simulink model "ModelStepper"  (R2020b)
settings: Solver=FixedStepAuto  StartTime=0.0  StopTime=10.0  FixedStep=0.010  RelTol=1e-3
settings Model: Creator=kaebi  LastModifiedBy=kaebi
settings ConfigComp: PLC_TargetIDE=codesys23

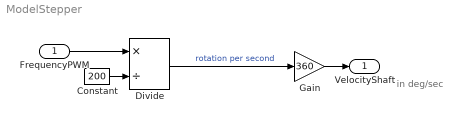
== system ModelStepper ==
  note: in deg/sec
  FrequencyPWM : Inport
  Constant : Constant  Value=200
  Divide : Product  Inputs=*/
  Gain : Gain  Gain=360
  VelocityShaft : Outport
  wires:
  FrequencyPWM/1 -> Divide/1
  Constant/1 -> Divide/2
  Divide/1 -> Gain/1  "rotation per second"
  Gain/1 -> VelocityShaft/1
